simulink model "q_qube2_ss_model_impulse"  (Simulink 8.3)
settings: Solver=ode1  StartTime=0.0  StopTime=inf  FixedStep=0.002  RelTol=1e-3
values from neighbouring files (symbols this model uses):
  A = [0 0 1 0 ... (first row only)    [QUBE2_ROTPEN_ABCD_eqns.m]    (also in rotpen_ABCD_eqns.m; setup_inverted_pend_ss_model.m; setup_non_inverted_pend_ss_model.m)
  B = kt * B / Rm    [QUBE2_ROTPEN_ABCD_eqns.m]    (also in rotpen_ABCD_eqns.m = km * B / Rm; setup_inverted_pend_ss_model.m; setup_non_inverted_pend_ss_model.m = km * B / Rm)
  C = eye(4,4)    [QUBE2_ROTPEN_ABCD_eqns.m]    (also in rotpen_ABCD_eqns.m = eye(2,4); setup_inverted_pend_ss_model.m; setup_non_inverted_pend_ss_model.m = eye(2,4))
  D = zeros(4,1)    [QUBE2_ROTPEN_ABCD_eqns.m]    (also in rotpen_ABCD_eqns.m = zeros(2,1); setup_inverted_pend_ss_model.m; setup_non_inverted_pend_ss_model.m = zeros(2,1))
undefined symbols (not defined in the file or in its folder): HIL, qc_get_step_size
libraries: quarc_library x3
settings Model: Creator=pmartin  LastModifiedBy=mbohra  SimulationMode=external  ExtModeTrigDuration=5000
settings SolverCC: PositivePriorityOrder=on
settings DataIOCC: SignalLoggingSaveFormat=Dataset
settings OptimizationCC: ExpressionDepthLimit=2147483647
settings DebuggingCC: FcnCallInpInsideContextMsg=EnableAllAsWarning
settings RTWCC: SystemTargetFile=quarc_win64.tlc  TemplateMakefile=quarc_default_tmf  Description=QUARC Win64 Target  ProcessScript=quarc_win64_make_rtw_hook
settings STFCustomTargetCC: TargetPreCompLibLocation=C:\PROGRA~3\QUARC\lib\2014a\win64\release  ConcurrentExecutionCompliant=on  GeneratePreprocessorConditionals=Disable all  CPPClassGenCompliant=on  SystemTargetFile=quarc_win64.tlc
settings GRTTargetCC: TargetPreCompLibLocation=C:\PROGRA~3\QUARC\lib\2014a\win64\release  ParMdlRefBuildCompliant=off  CompOptLevelCompliant=off  MatFileLogging=off  ExtMode=on  ExtModeMexFile=quarc_comm

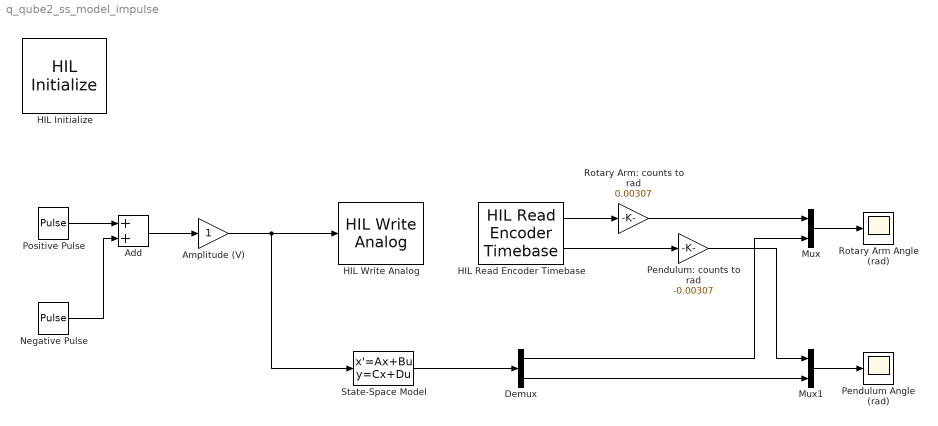
== system q_qube2_ss_model_impulse ==
  Add : Sum
  Amplitude (V) : Gain
  Demux : Demux  Outputs=2
  HIL Initialize : quarc_library/Data Acquisition/Generic/Configuration/HIL Initialize  Priority=-99  object_name=HIL-1  board_type=qube_servo2_usb  board_number=0  board_options=""  exclusive=off  active=off  hardware_clocks=[0]  clock_modes=[]  initial_clock_frequencies=[]  set_clock_params_at_start=off  set_clock_params_at_switch_in=off  set_clock_frequencies_at_start=off  set_clock_frequencies_at_switch_in=off  analog_input_channels=[0]  analog_input_maximums=3  analog_input_minimums=-3  set_analog_input_params_at_start=off  set_analog_input_params_at_switch_in=off  analog_output_channels=[0]  analog_output_maximums=15  analog_output_minimums=-15  initial_analog_outputs=[0]  final_analog_outputs=[0]  watchdog_analog_outputs=0  set_analog_output_params_at_start=off  set_analog_output_params_at_switch_in=off  set_analog_outputs_at_start=on  set_analog_outputs_at_switch_in=off  set_analog_outputs_at_terminate=on  set_analog_outputs_at_switch_out=off  set_analog_outputs_on_watchdog=on  digital_input_channels=[]  digital_output_channels=[0]  digital_output_configuration=[]  initial_digital_outputs=[1]  final_digital_outputs=[0]  watchdog_digital_outputs=[0]  set_digital_output_params_at_start=off  set_digital_output_params_at_switch_in=off  set_digital_outputs_at_start=on  set_digital_outputs_at_switch_in=off  set_digital_outputs_at_terminate=on  set_digital_outputs_at_switch_out=off  set_digital_outputs_on_watchdog=on  encoder_channels=[0:1]  quadrature=[4]  encoder_filter_frequency=[]  initial_encoder_counts=[0]  set_encoder_params_at_start=off  set_encoder_params_at_switch_in=off  set_encoder_counts_at_start=on  set_encoder_counts_at_switch_in=off  pwm_channels=[]  pwm_modes=[]  pwm_frequency=[]  pwm_configuration=[]  pwm_alignment=[]  pwm_polarity=[]  pwm_leading_deadband=[]  pwm_trailing_deadband=[]  initial_pwm_outputs=[]  final_pwm_outputs=[]  watchdog_pwm_outputs=[]  set_pwm_params_at_start=off  set_pwm_params_at_switch_in=off  set_pwm_outputs_at_start=off  set_pwm_outputs_at_switch_in=off  set_pwm_outputs_at_terminate=off  set_pwm_outputs_at_switch_out=off  set_pwm_outputs_on_watchdog=off  other_output_channels=[11000:11002]  initial_other_outputs=[0 1 0]  final_other_outputs=[1 0 0]  watchdog_other_outputs=[0 0 1]  set_other_outputs_at_start=on  set_other_outputs_at_switch_in=off  set_other_outputs_at_terminate=on  set_other_outputs_at_switch_out=off  set_other_outputs_on_watchdog=on
  HIL Read Encoder Timebase : quarc_library/Data Acquisition/Generic/Timebases/HIL Read Encoder Timebase  object_name=HIL-1  clock=0  channels=[0,1]  samples_in_buffer=max(ceil(1/qc_get_step_size), 1)  active=on  vector_output=off  data_type_mode=Inherit via back propagation  data_type=double
  HIL Write Analog : quarc_library/Data Acquisition/Generic/Immediate I//O/HIL Write Analog  object_name=HIL-1  channels=0  sample_time=-1  active=off  vector_input=off
  Mux : Mux  Inputs=2
  Mux1 : Mux  Inputs=2
  Negative Pulse : DiscretePulseGenerator  PulseType=Time based  Amplitude=-1  Period=4  PulseWidth=5  PhaseDelay=2
  Pendulum Angle (rad) : Scope
      settings: YMin=-0.3  YMax=0.275
  Pendulum: counts to rad : Gain  Gain=-0.00307
  Positive Pulse : DiscretePulseGenerator  PulseType=Time based  Period=4  PulseWidth=5
  Rotary Arm Angle (rad) : Scope
      settings: YMin=-1  YMax=0.9
  Rotary Arm: counts to rad : Gain  Gain=0.00307
  State-Space Model : StateSpace  A=A  B=B  C=C  D=D  X0=[0 0 0 0]
  wires:
  Amplitude (V)/1 -> HIL Write Analog/1, State-Space Model/1
  State-Space Model/1 -> Demux/1
  HIL Read Encoder Timebase/1 -> Rotary Arm: counts to rad/1
  Mux/1 -> Rotary Arm Angle (rad)/1
  Demux/1 -> Mux/2
  HIL Read Encoder Timebase/2 -> Pendulum: counts to rad/1
  Demux/2 -> Mux1/2
  Mux1/1 -> Pendulum Angle (rad)/1
  Rotary Arm: counts to rad/1 -> Mux/1
  Pendulum: counts to rad/1 -> Mux1/1
  Add/1 -> Amplitude (V)/1
  Positive Pulse/1 -> Add/1
  Negative Pulse/1 -> Add/2
